simulink model "KaskadeControlled"  (R2013a)
settings: Solver=ode1  StartTime=0.0  StopTime=Tend  FixedStep=Tstep  MaxStep=0.01  RelTol=1e-3
PreLoadFcn:
  | run KaskadeModellInit
values from neighbouring files (symbols this model uses):
  alphamax = 20/360*2*pi    (= 0.349065850399)    [KaskadeModellInit.m]
  alphapmax = 30/360*2*pi    (= 0.523598775598)    [KaskadeModellInit.m]
settings Model: Creator=Amann  LastModifiedBy=akuhenn
settings SolverCC: InitialStep=0.01

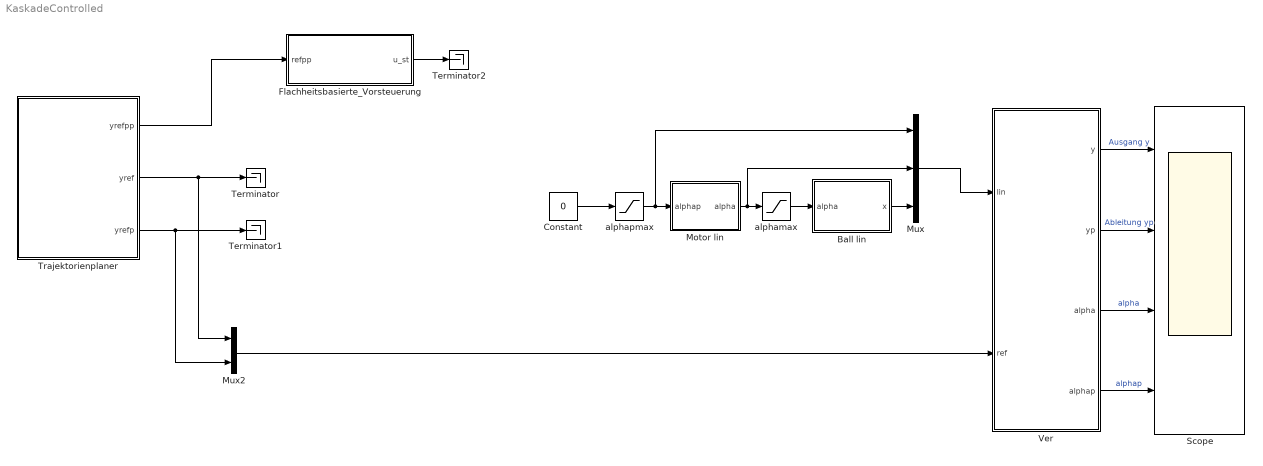
== system KaskadeControlled ==
  Ball lin : Subsystem
  Constant : Constant  Value=0
  Flachheitsbasierte_Vorsteuerung : Subsystem
  Motor lin : Subsystem
  Mux : Mux  Inputs=3
  Mux2 : Mux  Inputs=2
  Scope : Scope  NumInputPorts=4
      settings: YMin=-5~-5~-5~-5  YMax=5~5~5~5
  Terminator : Terminator
  Terminator1 : Terminator
  Terminator2 : Terminator
  Trajektorienplaner : Subsystem
  Ver : Subsystem
  alphamax : Saturate  UpperLimit=alphamax  LowerLimit=-alphamax
  alphapmax : Saturate  UpperLimit=alphapmax  LowerLimit=-alphapmax
  wires:
  Ver/1(y) -> Scope/1  "Ausgang y"
  Ver/2(yp) -> Scope/2  "Ableitung yp"
  Ver/3(alpha) -> Scope/3  "alpha"
  Motor lin/1(alpha) -> alphamax/1, Mux/2
  Ball lin/1(x) -> Mux/3
  Trajektorienplaner/3(yrefp) -> Terminator1/1, Mux2/2
  Trajektorienplaner/2(yref) -> Mux2/1, Terminator/1
  Mux/1 -> Ver/1(lin)
  Mux2/1 -> Ver/2(ref)
  Ver/4(alphap) -> Scope/4  "alphap"
  Constant/1 -> alphapmax/1
  alphapmax/1 -> Mux/1, Motor lin/1(alphap)
  alphamax/1 -> Ball lin/1(alpha)
  Trajektorienplaner/1(yrefpp) -> Flachheitsbasierte_Vorsteuerung/1(refpp)
  Flachheitsbasierte_Vorsteuerung/1(u_st) -> Terminator2/1

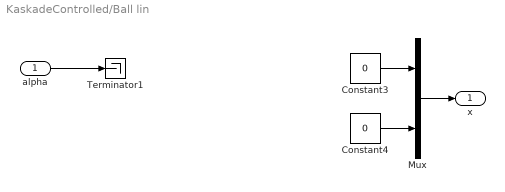
== system KaskadeControlled/Ball lin ==
  alpha : Inport
  Constant3 : Constant  Value=0
  Constant4 : Constant  Value=0
  Mux : Mux  Inputs=2
  Terminator1 : Terminator
  x : Outport
  wires:
  Mux/1 -> x/1
  Constant4/1 -> Mux/2
  Constant3/1 -> Mux/1
  alpha/1 -> Terminator1/1

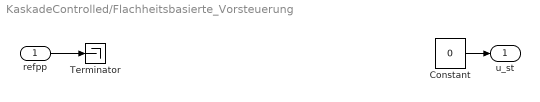
== system KaskadeControlled/Flachheitsbasierte_Vorsteuerung ==
  refpp : Inport
  Constant : Constant  Value=0
  Terminator : Terminator
  u_st : Outport
  wires:
  refpp/1 -> Terminator/1
  Constant/1 -> u_st/1

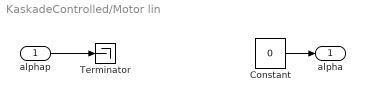
== system KaskadeControlled/Motor lin ==
  alphap : Inport
  Constant : Constant  Value=0
  Terminator : Terminator
  alpha : Outport
  wires:
  alphap/1 -> Terminator/1
  Constant/1 -> alpha/1

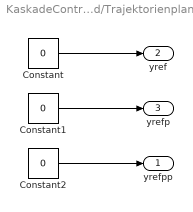
== system KaskadeControlled/Trajektorienplaner ==
  Constant : Constant  Value=0
  Constant1 : Constant  Value=0
  Constant2 : Constant  Value=0
  yrefpp : Outport
  yref : Outport  Port=2
  yrefp : Outport  Port=3
  wires:
  Constant/1 -> yref/1
  Constant1/1 -> yrefp/1
  Constant2/1 -> yrefpp/1

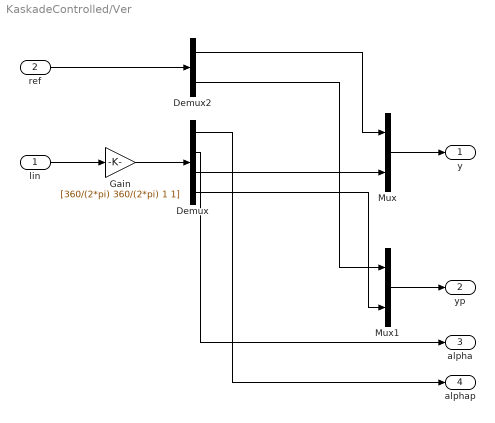
== system KaskadeControlled/Ver ==
  lin : Inport
  ref : Inport  Port=2
  Demux : Demux
  Demux2 : Demux  Outputs=2
  Gain : Gain  Gain=[360/(2*pi) 360/(2*pi) 1 1]
  Mux : Mux  Inputs=2
  Mux1 : Mux  Inputs=2
  y : Outport
  yp : Outport  Port=2
  alpha : Outport  Port=3
  alphap : Outport  Port=4
  wires:
  lin/1 -> Gain/1
  Gain/1 -> Demux/1
  Mux/1 -> y/1
  Demux/2 -> alpha/1
  ref/1 -> Demux2/1
  Mux1/1 -> yp/1
  Demux/1 -> alphap/1
  Demux2/1 -> Mux/1
  Demux2/2 -> Mux1/1
  Demux/3 -> Mux/2
  Demux/4 -> Mux1/2
